simulink model "voice_link_lms_channel_timeseries_system"  (R2026a)
settings: Solver=FixedStepDiscrete  StopTime=1  FixedStep=1
settings Model: Creator=24470  LastModifiedBy=24470

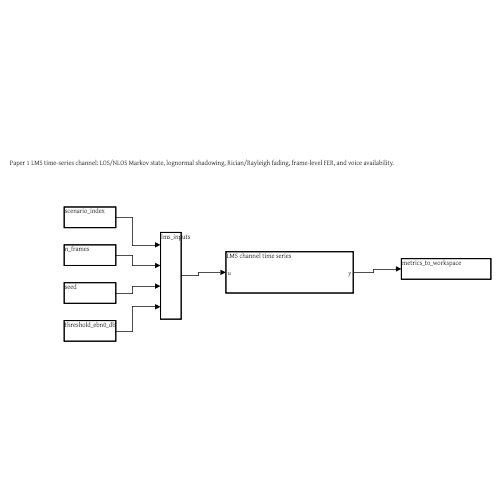
[thumbnail: Simulink's stored preview of the top-level diagram]
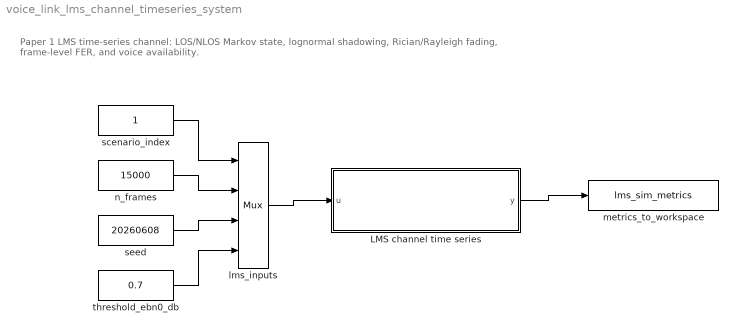
== system voice_link_lms_channel_timeseries_system ==
  note: Paper 1 LMS time-series channel: LOS/NLOS Markov state, lognormal shadowing, Rician/Rayleigh fading, frame-level FER, and voice availability.
  LMS channel time series : MATLAB Function  TreatAsAtomicUnit=on
  lms_inputs : Mux
  metrics_to_workspace : ToWorkspace  VariableName=lms_sim_metrics  SampleTime=-1
  n_frames : Constant  Value=15000
  scenario_index : Constant
  seed : Constant  Value=20260608
  threshold_ebn0_db : Constant  Value=0.7
  wires:
  scenario_index/1 -> lms_inputs/1
  n_frames/1 -> lms_inputs/2
  seed/1 -> lms_inputs/3
  threshold_ebn0_db/1 -> lms_inputs/4
  lms_inputs/1 -> LMS channel time series/1(u)
  LMS channel time series/1(y) -> metrics_to_workspace/1

== matlab function voice_link_lms_channel_timeseries_system/LMS channel time series ==
  data: u input; y output
function y = fcn(u)
%#codegen
coder.extrinsic('paper1_simulink_lms_scenario');
y = zeros(9,1);
y = paper1_simulink_lms_scenario(u);
end
